simulink model "demo1"  (R2019a)
settings: Solver=VariableStepAuto  StartTime=0.0  StopTime=10.0  RelTol=1e-3
libraries: simulink x1
settings Model: Creator=chute  LastModifiedBy=chute

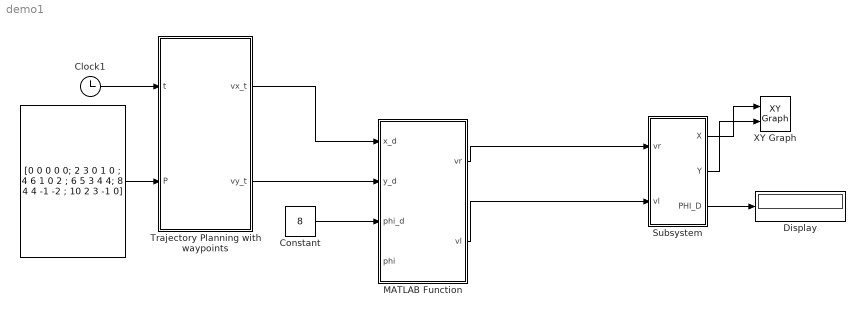
== system demo1 ==
  " " : Constant  Value=[0 0 0 0 0; 2 3 0 1 0 ; 4 6 1 0 2 ; 6 5 3 4 4; 8 4 4 -1 -2 ; 10 2 3 -1 0]  VectorParams1D=off  SampleTime=-1
  Clock1 : Clock
  Constant : Constant  Value=8
  Display : Display
  MATLAB Function : MATLAB Function  TreatAsAtomicUnit=on
  Subsystem : Subsystem
  Trajectory Planning with waypoints : MATLAB Function  TreatAsAtomicUnit=on
  XY Graph : simulink/Sinks/XY Graph  xmin=-1  xmax=20  ymin=-1  ymax=20  st=-1
  wires:
  MATLAB Function/1(vr) -> Subsystem/1(vr)
  MATLAB Function/2(vl) -> Subsystem/2("vl ")
  Constant/1 -> MATLAB Function/3(phi_d)
  Subsystem/3(PHI_D) -> Display/1
  Clock1/1 -> Trajectory Planning with waypoints/1(t)
  " "/1 -> Trajectory Planning with waypoints/2(P)
  Trajectory Planning with waypoints/2(vy_t) -> MATLAB Function/2(y_d)
  Trajectory Planning with waypoints/1(vx_t) -> MATLAB Function/1(x_d)
  Subsystem/1(X) -> XY Graph/1
  Subsystem/2(Y) -> XY Graph/2

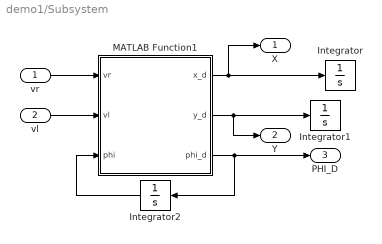
== system demo1/Subsystem ==
  vr : Inport
  "vl " : Inport  Port=2
  Integrator : Integrator
  Integrator1 : Integrator
  Integrator2 : Integrator
  MATLAB Function1 : MATLAB Function  TreatAsAtomicUnit=on
  X : Outport
  Y : Outport  Port=2
  PHI_D : Outport  Port=3
  wires:
  MATLAB Function1/1(x_d) -> X/1, Integrator/1
  vr/1 -> MATLAB Function1/1(vr)
  MATLAB Function1/2(y_d) -> Y/1, Integrator1/1
  "vl "/1 -> MATLAB Function1/2(vl)
  MATLAB Function1/3(phi_d) -> PHI_D/1, Integrator2/1
  Integrator2/1 -> MATLAB Function1/3(phi)

== matlab function demo1/Subsystem/MATLAB Function1 ==
  data: vr input; x_d output; vl input; y_d output; phi_d output; phi input
function [x_d,y_d,phi_d] = fcn(vr,vl,phi)
R=5;
W=2;
% Pesudo jacobian matrix
x_d=(R/2)*(vr*cos(phi)+vl*cos(phi));
y_d=(R/2)*(vr*sin(phi)+vl*sin(phi));
phi_d=(R/W)*(vr-vl);
end

== matlab function demo1/MATLAB Function ==
  data: x_d input; vr output; y_d input; phi_d input; phi input; vl output
function [vr,vl] = fcn(x_d,y_d,phi_d,phi)
R=5;
W=2;
% Pesudo jacobian matrix
vr=(1/R)*(x_d*cos(phi)+y_d*sin(phi)+(W/2)*phi_d);
vl=(1/R)*(x_d*cos(phi)+y_d*sin(phi)+(W/2)*phi_d);
end

== matlab function demo1/Trajectory Planning with waypoints ==
  data: t input; vx_t output; vy_t output; P input
function [vx_t,vy_t] = fcn(t,P)
%% Quy hoach quy dao
k = size(P,1)-1;                                        % So giai doan chay, i diem thi i-1 giai doan
ai = zeros(k,8);                                        % Ma tran K*8 luu cac gia tri a0-a4 cua X,Y
for i=1:k
    ai(i,:) = Trajectory_Planning(P(i,:),P(i+1,:));     % Tinh gia tri a0-a4 doi voi tung diem P(x,y)
end
%% Xuat quy dao
ti = P(2,1);                                            % Thoi gian lay mau giua 2 diem
if(t<P(k+1,1))
    j = floor(t/ti)+1;                                  % Xac dinh giai doan hien tai cua quy dao
    vx_t = ai(j,2) + 2*ai(j,3)*t + 3*ai(j,4)*t^2;
    vy_t = ai(j,6) + 2*ai(j,7)*t + 3*ai(j,8)*t^2;
else
    vx_t = P(k+1,4);
    vy_t = P(k+1,5);
end
end
